simulink library "scddemolib"  (Simulink 7.6)
settings: Solver=ode45  SolverMode=SingleTasking  StartTime=0.0  StopTime=10.0  RelTol=1e-3
settings Model: Creator=The MathWorks Inc.

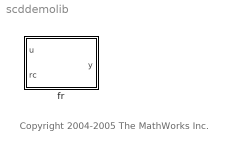
== system scddemolib ==
  note: Copyright 2004-2005 The MathWorks Inc.
  fr : Stateflow chart  TreatAsAtomicUnit=on

== matlab function fr ==
  data: u input double size=1; y output double size=1; rc input double size=1
function y = fcn(u, rc)

gam = 1.4;

if u > 1
    y = 0;
elseif u >= rc
    y = sqrt(2*gam/(gam-1))*sqrt(u^(2/gam)-u^((gam+1)/gam));
else
    y = sqrt(gam*(2/(gam+1))^((gam+1)/(gam-1)));
end
